simulink model "MPC_PlanCtrl"  (R2022b)
settings: Solver=VariableStepDiscrete  StartTime=0.0  StopTime=36  FixedStep=0.01  RelTol=1e-3  EnableMultiTasking=on
libraries: Solver_SF x1
settings Model: Creator=xuwei  LastModifiedBy=wyx
settings SolverCC: AlgebraicLoopSolver=TrustRegion
settings DataIOCC: LimitDataPoints=on  SaveFormat=Array  SignalLoggingSaveFormat=ModelDataLogs  ReturnWorkspaceOutputs=off
settings OptimizationCC: ExpressionDepthLimit=2147483647  LifeSpan=inf
settings DebuggingCC: UnderspecifiedInitializationDetection=Classic  MergeDetectMultiDrivingBlocksExec=none  SolverPrmCheckMsg=warning  FcnCallInpInsideContextMsg=warning  UnconnectedInputMsg=warning  UnconnectedOutputMsg=warning  UnconnectedLineMsg=warning  StateNameClashWarn=warning  SFUnexpectedBacktrackingDiag=warning  SFNoUnconditionalDefaultTransitionDiag=warning  SFExecutionAtInitializationDiag=none  SFMachineParentedDataDiag=warning  ArithmeticOperatorsInVariantConditions=warning
settings HardwareCC: ProdBitPerPointer=32  ProdBitPerSizeT=32  ProdBitPerPtrDiffT=32  ProdLargestAtomicFloat=None  ProdIntDivRoundTo=Undefined  ProdEndianess=Unspecified  ProdWordSize=32  ProdHWDeviceType=32-bit Generic
settings ModelReferenceCC: PropagateSignalLabelsOutOfModel=off
settings SFSimCC: SimUseLocalCustomCode=off  CustomCodeUndefinedFunction=UseInterfaceOnly
settings RTWCC: RTWUseLocalCustomCode=off
settings CodeAppCC: StateflowObjectComments=on
settings GRTTargetCC: TargetLangStandard=C89/C90 (ANSI)  CombineOutputUpdateFcns=off  GRTInterface=on
settings ConfigComp: CovMetricSettings=dw  CovSaveCumulativeToWorkspaceVar=on  CovSaveSingleToWorkspaceVar=on  CovExternalEMLEnable=off

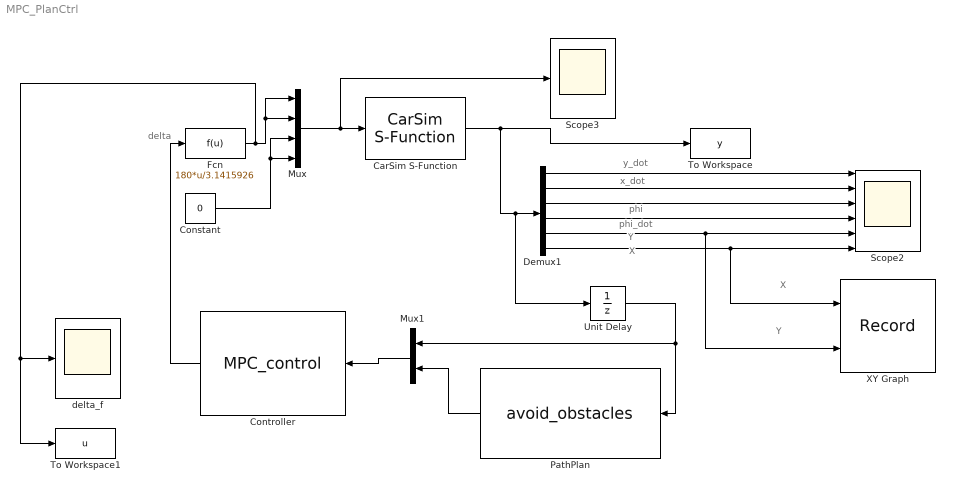
== system MPC_PlanCtrl ==
  note: delta
  note: X
  note: Y
  note: y_dot
  note: x_dot
  note: phi
  note: phi_dot
  note: Y
  note: X
  CarSim S-Function : Solver_SF/CarSim S-Function  Priority=1  SIMFILE=simfile.sim
  Constant : Constant  Value=0
  Controller : S-Function  FunctionName=MPC_control  SFunctionDeploymentMode=off  EnableBusSupport=off
  Demux1 : Demux  Outputs=6
  Fcn : Fcn  Expr=180*u/3.1415926
  Mux : Mux
  Mux1 : Mux  Inputs=2
  PathPlan : S-Function  FunctionName=avoid_obstacles  SFunctionDeploymentMode=off  EnableBusSupport=off
  Scope2 : Scope  NumInputPorts=6
  Scope3 : Scope
  To Workspace : ToWorkspace  VariableName=y  SaveFormat=Structure  SampleTime=-1
  To Workspace1 : ToWorkspace  VariableName=u  SaveFormat=Structure  SampleTime=-1
  Unit Delay : UnitDelay  SampleTime=-1  HasFrameUpgradeWarning=on
  XY Graph : Record  FileSettingsInternal="{\"entries\":[{\"content\":{\"excelSettings\":{\"content\":{},\"type\":\"Streamout.ExcelSettings\"}},\"type\":\"Streamout.FileSettingStorage\",\"uuid\":\"324f603e-1c90-46e0-a459-460468ca5ad6\"}],\"packageUris\":[\"http://schema.mathworks.com/mf0/streamout_blocks/R2020a\"],\"version\":\"1.0\"}"  Layout=[1 1]  SignalsInternal="{\"entries\":[{\"content\":{\"signals\":[{\"content\":{\"blockPath\":[\"MPC_PlanCtrl/XY Graph\"],\"channel\":[],\"dimensions\":[1],\"domain\":\"MPC_PlanCtrl/XY Graph\",\"lineColor\":\"#a2142f\",\"plots\":[1],\"port\":1,\"sid\":[\"\"],\"signalID\":2141,\"signalName\":\"Demux1:6\"},\"type\":\"RecordBlkView.Signal\",\"uuid\":\"38146ec6-851b-4b07-879b-ec553731f642\"},{\"content\":{\"blockPath\":[\"MPC_PlanCtrl/XY Graph\"],\"channel\":[],\"dimensions\":[1],\"domain\":\"MPC_PlanCtrl/XY Graph\",\"lineColor\":\"#139fff\",\"plots\":[1],\"port\":2,\"sid\":[\"\"],\"signalID\":2145,\"signalName\":\"Demux1:5\"},\"type\":\"RecordBlkView.Signal\",\"uuid\":\"e2c6fc05-2cf0-48dd-a851-236654742e7d\"}]},\"type\":\"RecordBlkView.InputSignals\",\"uuid\":\"a60e4577-95ef-4084-93ad-1253e870e3dc\"}],\"packageUris\":[\"http://schema.mathworks.com/mf0/streamout_blocks/R2020a\"],\"version\":\"1.0\"}"  VisualizationBindings="{\"xyplotplugin\":{\"info\":[{\"series\":[{\"bindingParametersList\":[{\"parameter\":\"X-Axis\",\"signalID\":2141,\"signalName\":\"Demux1:6\"},{\"parameter\":\"Y-Axis\",\"signalID\":2145,\"signalName\":\"Demux1:5\"}],\"seriesID\":19299}],\"subplotID\":1}]}}"  CompatibilityTag=XY  st=-1
  delta_f : Scope
  wires:
  CarSim S-Function/1 -> To Workspace/1, Demux1/1, Unit Delay/1
  Fcn/1 -> Mux/1, Mux/2, delta_f/1, To Workspace1/1
  Constant/1 -> Mux/4, Mux/3
  Mux/1 -> CarSim S-Function/1, Scope3/1
  Demux1/1 -> Scope2/1
  Demux1/2 -> Scope2/2
  Demux1/3 -> Scope2/3
  Demux1/4 -> Scope2/4
  Demux1/5 -> Scope2/5, XY Graph/2
  Demux1/6 -> Scope2/6, XY Graph/1
  Controller/1 -> Fcn/1
  Unit Delay/1 -> Mux1/1, PathPlan/1
  PathPlan/1 -> Mux1/2
  Mux1/1 -> Controller/1
